simulink model "mtrigport_noio"  (Simulink 8.0)
settings: Solver=FixedStepDiscrete  StartTime=0.0  StopTime=10.0  FixedStep=1  RelTol=1e-3
settings Model: Creator=mtocci  LastModifiedBy=mtocci
settings DataIOCC: LimitDataPoints=off  SaveFormat=StructureWithTime  SignalLoggingSaveFormat=ModelDataLogs
settings OptimizationCC: InlineParams=on
settings DebuggingCC: FcnCallInpInsideContextMsg=Use local settings  StrictBusMsg=ErrorOnBusTreatedAsVector
settings GRTTargetCC: CombineOutputUpdateFcns=off

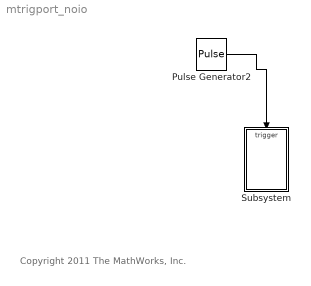
== system mtrigport_noio ==
  note: Copyright 2011 The MathWorks, Inc.
  Pulse Generator2 : DiscretePulseGenerator  Amplitude=[1 1 2 2]
  Subsystem : Subsystem
  wires:
  Pulse Generator2/1 -> Subsystem/Trigger

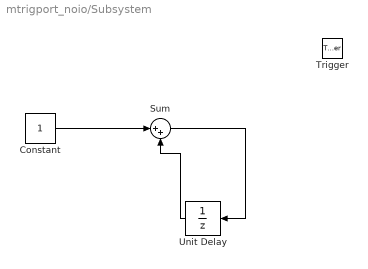
== system mtrigport_noio/Subsystem ==
  Trigger : TriggerPort  PortDimensions=1
  Constant : Constant
  Sum : Sum  Inputs=|++
  Unit Delay : UnitDelay  SampleTime=-1
  wires:
  Sum/1 -> Unit Delay/1
  Unit Delay/1 -> Sum/2
  Constant/1 -> Sum/1
